simulink model "fullSim"  (R2015b)
settings: Solver=VariableStepAuto  StartTime=0.0  StopTime=1  RelTol=1e-3
settings Model: Creator=Ricardo  LastModifiedBy=Ricardo

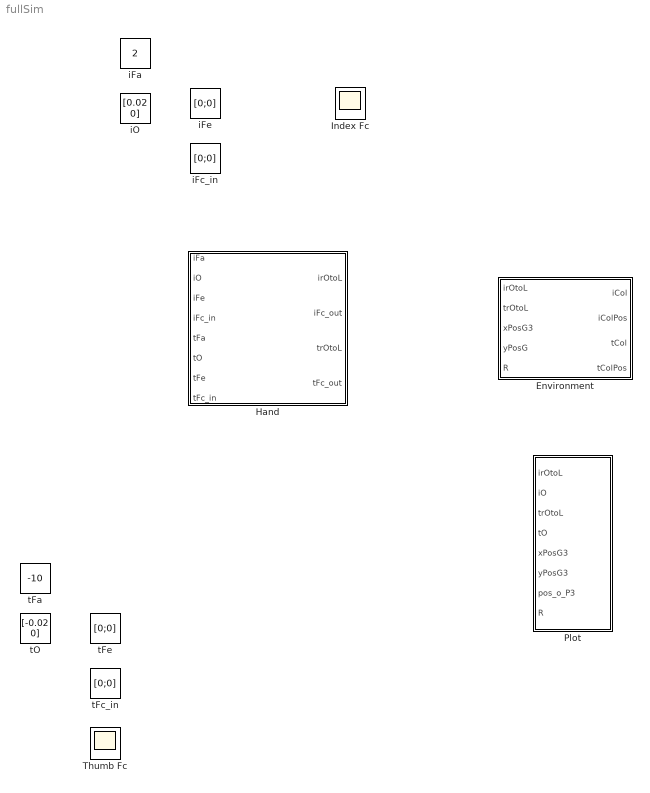
== system fullSim ==
  Environment : Subsystem
  Hand : Subsystem
  Index Fc : Scope
  Plot : Subsystem
  Thumb Fc : Scope
  iFa : Constant  Value=2
  iFc_in : Constant  Value=[0;0]
  iFe : Constant  Value=[0;0]
  iO : Constant  Value=[0.02 0]
  tFa : Constant  Value=-10
  tFc_in : Constant  Value=[0;0]
  tFe : Constant  Value=[0;0]
  tO : Constant  Value=[-0.02 0]

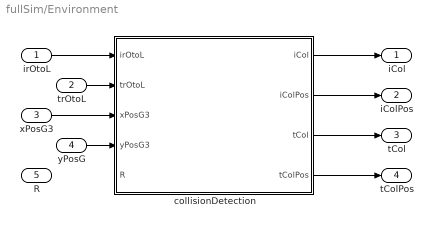
== system fullSim/Environment ==
  irOtoL : Inport
  trOtoL : Inport  Port=2
  xPosG3 : Inport  Port=3
  yPosG : Inport  Port=4
  R : Inport  Port=5
  collisionDetection : MATLAB Function  TreatAsAtomicUnit=on
  iCol : Outport
  iColPos : Outport  Port=2
  tCol : Outport  Port=3
  tColPos : Outport  Port=4
  wires:
  trOtoL/1 -> collisionDetection/2(trOtoL)
  irOtoL/1 -> collisionDetection/1(irOtoL)
  xPosG3/1 -> collisionDetection/3(xPosG3)
  yPosG/1 -> collisionDetection/4(yPosG3)
  collisionDetection/1(iCol) -> iCol/1
  collisionDetection/4(tColPos) -> tColPos/1
  collisionDetection/3(tCol) -> tCol/1
  collisionDetection/2(iColPos) -> iColPos/1

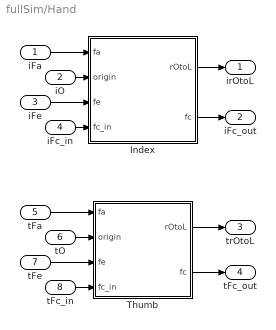
== system fullSim/Hand ==
  iFa : Inport
  iO : Inport  Port=2
  iFe : Inport  Port=3
  iFc_in : Inport  Port=4
  tFa : Inport  Port=5
  tO : Inport  Port=6
  tFe : Inport  Port=7
  tFc_in : Inport  Port=8
  Index : Subsystem
  Thumb : Subsystem
  irOtoL : Outport
  iFc_out : Outport  Port=2
  trOtoL : Outport  Port=3
  tFc_out : Outport  Port=4
  wires:
  iFa/1 -> Index/1(fa)
  iO/1 -> Index/2(origin)
  iFe/1 -> Index/3(fe)
  iFc_in/1 -> Index/4(fc_in)
  Index/1(rOtoL) -> irOtoL/1
  Index/2(fc) -> iFc_out/1
  tFa/1 -> Thumb/1(fa)
  tO/1 -> Thumb/2(origin)
  tFe/1 -> Thumb/3(fe)
  tFc_in/1 -> Thumb/4(fc_in)
  Thumb/1(rOtoL) -> trOtoL/1
  Thumb/2(fc) -> tFc_out/1

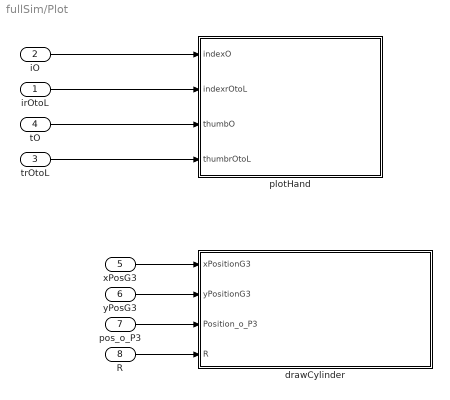
== system fullSim/Plot ==
  irOtoL : Inport
  iO : Inport  Port=2
  trOtoL : Inport  Port=3
  tO : Inport  Port=4
  xPosG3 : Inport  Port=5
  yPosG3 : Inport  Port=6
  pos_o_P3 : Inport  Port=7
  R : Inport  Port=8
  drawCylinder : MATLAB Function  TreatAsAtomicUnit=on
  plotHand : MATLAB Function  TreatAsAtomicUnit=on
  wires:
  iO/1 -> plotHand/1(indexO)
  tO/1 -> plotHand/3(thumbO)
  irOtoL/1 -> plotHand/2(indexrOtoL)
  trOtoL/1 -> plotHand/4(thumbrOtoL)
  xPosG3/1 -> drawCylinder/1(xPositionG3)
  yPosG3/1 -> drawCylinder/2(yPositionG3)
  pos_o_P3/1 -> drawCylinder/3(Position_o_P3)
  R/1 -> drawCylinder/4(R)

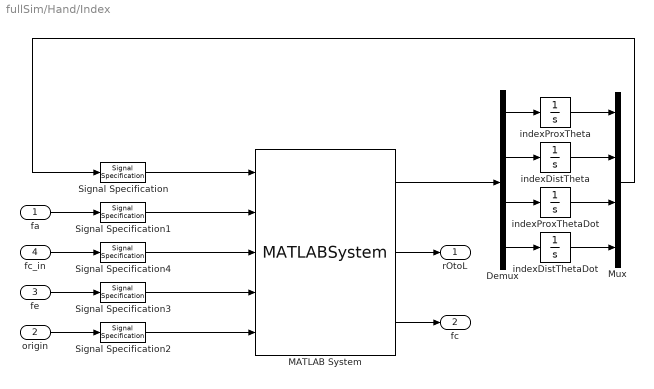
== system fullSim/Hand/Index ==
  fa : Inport
  origin : Inport  Port=2
  fe : Inport  Port=3
  fc_in : Inport  Port=4
  Demux : Demux
  MATLAB System : MATLABSystem  System=Index  kP=-0.043  kD=-0.185  dP=-0.01  dD=-0.01  lP=0.1  lD=0.1  rP=0.02  rD=0.012  mP=0.02  mD=0.02  thetaP=pi/10  thetaD=pi/3  SimulateUsing=Interpreted execution
      mask Type: Index
      mask Display:
      | disp('Index');
      | port_label('input',1,'initVal');
      | port_label('input',2,'fa');
      | port_label('input',3,'fc');
      | port_label('input',4,'fe');
      | port_label('input',5,'origin');
      | port_label('output',1,'xDot');
      | port_label('output',2,'rOtoL');
      | port_label('output',3,'fc');
  Mux : Mux
  Signal Specification : SignalSpecification  Dimensions=4
  Signal Specification1 : SignalSpecification  Dimensions=1
  Signal Specification2 : SignalSpecification  Dimensions=2
  Signal Specification3 : SignalSpecification  Dimensions=2
  Signal Specification4 : SignalSpecification  Dimensions=2
  indexDistTheta : Integrator  InitialCondition=pi/3  ContinuousStateAttributes='indexDistTheta'
  indexDistThetaDot : Integrator  ContinuousStateAttributes='indexDistThetaDot'
  indexProxTheta : Integrator  InitialCondition=pi/10  ContinuousStateAttributes='indexProxTheta'
  indexProxThetaDot : Integrator  ContinuousStateAttributes='indexProxThetaDot'
  rOtoL : Outport
  fc : Outport  Port=2
  wires:
  Demux/1 -> indexProxTheta/1
  Demux/2 -> indexDistTheta/1
  Demux/3 -> indexProxThetaDot/1
  Demux/4 -> indexDistThetaDot/1
  MATLAB System/1 -> Demux/1
  indexProxTheta/1 -> Mux/1
  indexDistTheta/1 -> Mux/2
  indexProxThetaDot/1 -> Mux/3
  indexDistThetaDot/1 -> Mux/4
  Mux/1 -> Signal Specification/1
  Signal Specification/1 -> MATLAB System/1
  MATLAB System/2 -> rOtoL/1
  MATLAB System/3 -> fc/1
  Signal Specification1/1 -> MATLAB System/2
  fa/1 -> Signal Specification1/1
  origin/1 -> Signal Specification2/1
  Signal Specification2/1 -> MATLAB System/5
  fe/1 -> Signal Specification3/1
  Signal Specification3/1 -> MATLAB System/4
  fc_in/1 -> Signal Specification4/1
  Signal Specification4/1 -> MATLAB System/3

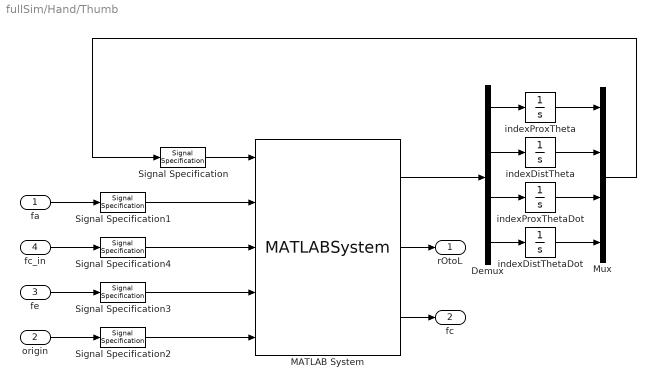
== system fullSim/Hand/Thumb ==
  fa : Inport
  origin : Inport  Port=2
  fe : Inport  Port=3
  fc_in : Inport  Port=4
  Demux : Demux
  MATLAB System : MATLABSystem  System=Thumb  kP=-1  kD=-5  dP=-0.01  dD=-0.01  lP=0.1  lD=0.1  rP=0.02  rD=0.012  mP=0.02  mD=0.02  thetaP=pi-pi/10  thetaD=-pi/3  SimulateUsing=Interpreted execution
      mask Type: Thumb
      mask Display:
      | disp('Thumb');
      | port_label('input',1,'initVal');
      | port_label('input',2,'fa');
      | port_label('input',3,'fc');
      | port_label('input',4,'fe');
      | port_label('input',5,'origin');
      | port_label('output',1,'xDot');
      | port_label('output',2,'rOtoL');
      | port_label('output',3,'fc');
  Mux : Mux
  Signal Specification : SignalSpecification  Dimensions=4
  Signal Specification1 : SignalSpecification  Dimensions=1
  Signal Specification2 : SignalSpecification  Dimensions=2
  Signal Specification3 : SignalSpecification  Dimensions=2
  Signal Specification4 : SignalSpecification  Dimensions=2
  indexDistTheta : Integrator  InitialCondition=-pi/3  ContinuousStateAttributes='indexDistTheta'
  indexDistThetaDot : Integrator  ContinuousStateAttributes='indexDistThetaDot'
  indexProxTheta : Integrator  InitialCondition=pi-pi/10  ContinuousStateAttributes='indexProxTheta'
  indexProxThetaDot : Integrator  ContinuousStateAttributes='indexProxThetaDot'
  rOtoL : Outport
  fc : Outport  Port=2
  wires:
  Demux/1 -> indexProxTheta/1
  Demux/2 -> indexDistTheta/1
  Demux/3 -> indexProxThetaDot/1
  Demux/4 -> indexDistThetaDot/1
  MATLAB System/1 -> Demux/1
  fa/1 -> Signal Specification1/1
  indexProxTheta/1 -> Mux/1
  indexDistTheta/1 -> Mux/2
  indexProxThetaDot/1 -> Mux/3
  indexDistThetaDot/1 -> Mux/4
  Mux/1 -> Signal Specification/1
  Signal Specification/1 -> MATLAB System/1
  MATLAB System/2 -> rOtoL/1
  MATLAB System/3 -> fc/1
  origin/1 -> Signal Specification2/1
  fe/1 -> Signal Specification3/1
  Signal Specification3/1 -> MATLAB System/4
  fc_in/1 -> Signal Specification4/1
  Signal Specification4/1 -> MATLAB System/3
  Signal Specification1/1 -> MATLAB System/2
  Signal Specification2/1 -> MATLAB System/5

== matlab function fullSim/Environment/collisionDetection ==
  data: irOtoL input; iCol output; trOtoL input; xPosG3 input; yPosG3 input; R input; iColPos output; tCol output; tColPos output
% Handles collision detection between fingertips and Cylinder. 
% Handled in Simulink.
% Author: Ricardo Garcia Rosas
% Change log:
%%%%%%%%%%%%|%%%%%%%%%%%|%%%%%%%%%%%%%%%%%%%%%%%%%%%%%%%%%%%%%%%%%%%|
% Date      |   Author  | Notes                                     |
% 16/04/06  |   RGR     | Created.                                  |
function [iCol,iColPos,tCol,tColPos] = collisionDetection(irOtoL,trOtoL,xPosG3,yPosG3,R)
    % Handles collision detection between fingertips and Cylinder.
    % Performed by comparing object radius.
    
    % Get circle radius given object center and fingertip position.
    ri = sqrt((irOtoL(1,1)-xPosG3)^2+(irOtoL(2,1)-yPosG3)^2);
    ti = sqrt((trOtoL(1,1)-xPosG3)^2+(trOtoL(2,1)-yPosG3)^2);
    % Verify calculated radius with object radius to define collision.
    if(ri<=R)
        iCol = true;
        iColPos = irOtoL;
    else
        iCol = false;
        iColPos = [0;0];
    end
    if(ti<=R)
        tCol = true;
        tColPos = trOtoL;
    else
        tCol = false;
        tColPos = [0;0];
    end
    
end

== matlab function fullSim/Plot/plotHand ==
  data: indexO input; indexrOtoL input; thumbO input; thumbrOtoL input
% Plots the entire hand to the default figure. Handled in Simulink.
% Author: Ricardo Garcia Rosas
% Change log:
%%%%%%%%%%%%|%%%%%%%%%%%|%%%%%%%%%%%%%%%%%%%%%%%%%%%%%%%%%%%%%%%%%%%|
% Date      |   Author  | Notes                                     |
% 16/03/23  |   RGR     | Added more comments.                      |
function plotHand(indexO,indexrOtoL,thumbO,thumbrOtoL)
    % Plots the entire hand to the default figure. Handled in Simulink.
    % @param indexO Index finger origin position [x,y] (m).
    % @param indexrOtoL Index finger vector from its origin to its link
    % ends.
    % @param thumbO Thumb origin position [x,y] (m).
    % @param thumbrOtoL Thumb vector from its origin to its link ends.

    % Call figure
    figure(1);
    clf;
    hold on;
    % Draw pam
    plot([indexO(1) thumbO(1)],[indexO(2) thumbO(2)],'LineWidth',8,'Color', 'k');
    % Draw Proximal components of Index
    plot([indexO(1) indexrOtoL(1,1)],[indexO(2) indexrOtoL(2,1)],'LineWidth',8,'Color', 'k');
    plot(indexO(1),indexO(2),'ko','MarkerSize',18);
    % Draw Distal components of Index
    plot([indexrOtoL(1,1) indexrOtoL(1,2)],[indexrOtoL(2,1) indexrOtoL(2,2)],'LineWidth',8,'Color', 'k');
    plot(indexrOtoL(1,1),indexrOtoL(2,1),'ko','MarkerSize',18);
    % Draw Index fingertip
    plot(indexrOtoL(1,2),indexrOtoL(2,2),'ko','MarkerSize',8);
    % Draw Proximal components of Thumb
    plot([thumbO(1) thumbrOtoL(1,1)],[thumbO(2) thumbrOtoL(2,1)],'LineWidth',8,'Color', 'k');
    plot(thumbO(1),thumbO(2),'ko','MarkerSize',18);
    % Draw Distal components of Thumn
    plot([thumbrOtoL(1,1) thumbrOtoL(1,2)],[thumbrOtoL(2,1) thumbrOtoL(2,2)],'LineWidth',8,'Color', 'k');
    plot(thumbrOtoL(1,1),thumbrOtoL(2,1),'ko','MarkerSize',18);
    % Draw Thumb fingertip
    plot(thumbrOtoL(1,2),thumbrOtoL(2,2),'ko','MarkerSize',8);
    hold off;
    axis([-0.2 0.2 -0.05 0.2]);
end

== matlab function fullSim/Plot/drawCylinder ==
  data: xPositionG3 input; yPositionG3 input; Position_o_P3 input; R input
function DrawCylinder(xPositionG3,yPositionG3,Position_o_P3,R)
%#
    figure(2);
    clf;
    t=linspace(0,2*pi,360);
    plot(xPositionG3,yPositionG3,'r*');
    hold on
    plot(Position_o_P3(1),Position_o_P3(2),'r*');
    x=xPositionG3+R*cos(t);
    y=yPositionG3+R*sin(t);
    plot(x,y,'b');
    hold off
    axis([-0.4 0.4 -0.3 0.3]);
end
